simulink model "FM"  (R2021b)
settings: Solver=VariableStepAuto  StartTime=0.0  StopTime=5  RelTol=1e-3
libraries: commanapbnd3 x1
settings Model: Creator=user  LastModifiedBy=user

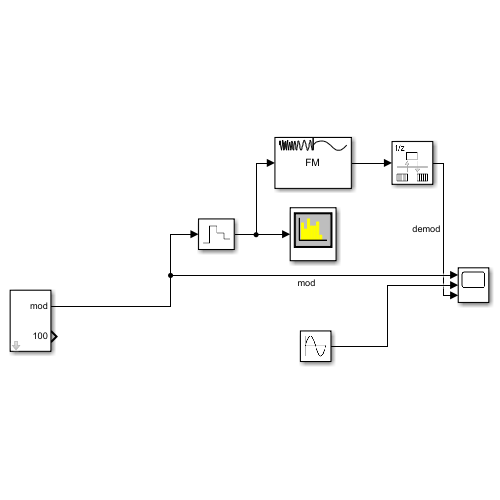
[thumbnail: Simulink's stored preview of the top-level diagram]
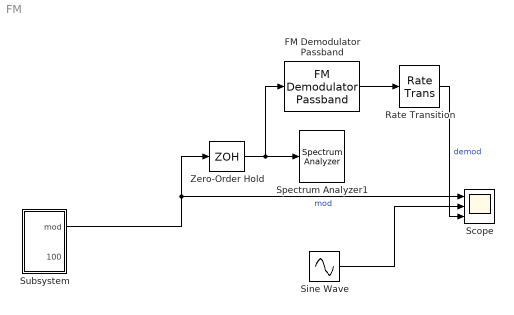
== system FM ==
  FM Demodulator Passband : commanapbnd3/FM Demodulator Passband  Fc=1000  Ph=0  Kc=500  Ho=100
      settings: SourceProductBaseCode=CM
  Rate Transition : RateTransition
  Scope : Scope  NumInputPorts=3
  Sine Wave : Sin  Frequency=100 * 2 * pi  SampleTime=0
  Spectrum Analyzer1 : SpectrumAnalyzer
  Subsystem : Subsystem  mask{d=1000}
      mask prompts: d "deviation"
  Zero-Order Hold : ZeroOrderHold  SampleTime=1e-4
  wires:
  Zero-Order Hold/1 -> FM Demodulator Passband/1, Spectrum Analyzer1/1
  Subsystem/1(mod) -> Zero-Order Hold/1, Scope/1  "mod"
  Rate Transition/1 -> Scope/3  "demod"
  FM Demodulator Passband/1 -> Rate Transition/1
  Sine Wave/1 -> Scope/2

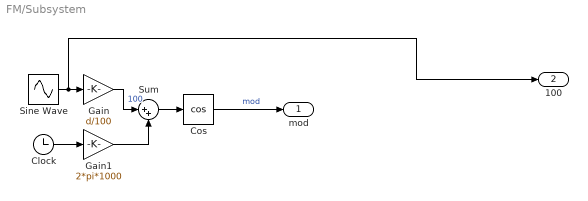
== system FM/Subsystem ==
  Clock : Clock
  Cos : Trigonometry  Operator=cos
  Gain : Gain  Gain=d/100
  Gain1 : Gain  Gain=2*pi*1000
  Sine Wave : Sin  Frequency=100 * 2 * pi  Phase=pi/2  SampleTime=0
  Sum : Sum  Inputs=|++
  mod : Outport
  100 : Outport  Port=2
  wires:
  Cos/1 -> mod/1  "mod"
  Sum/1 -> Cos/1
  Gain1/1 -> Sum/2
  Gain/1 -> Sum/1  "100"
  Sine Wave/1 -> 100/1, Gain/1
  Clock/1 -> Gain1/1
